simulink model "LE3_1"  (R2018a)
settings: Solver=ode4  StartTime=0.0  StopTime=10.0  FixedStep=0.001  RelTol=1e-3
settings Model: Creator=Kenneth  LastModifiedBy=Kenneth

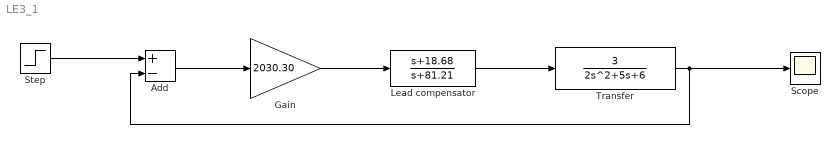
== system LE3_1 ==
  Add : Sum  Inputs=+-
  Gain : Gain  Gain=2030.30
  Lead compensator : TransferFcn  Numerator=[1 18.68]  Denominator=[1 81.21]
  Scope : Scope
  Step : Step  Time=0  Before=1  SampleTime=0
  Transfer : TransferFcn  Numerator=[3]  Denominator=[2 5 6]
  wires:
  Add/1 -> Gain/1
  Transfer/1 -> Scope/1, Add/2
  Lead compensator/1 -> Transfer/1
  Gain/1 -> Lead compensator/1
  Step/1 -> Add/1
